simulink subsystem "monocopterChassis"  (R2023a)
settings: Solver=VariableStepAuto  StartTime=0.0  StopTime=100  RelTol=1e-3
undefined symbols (not defined in the file): chassis, fixedStepSize, g
libraries: fl_lib x17, nesl_utility x4
settings Model: DefaultTestHarness=monocopterChassis_Harness1  Creator=imyrsini  LastModifiedBy=imyrsini

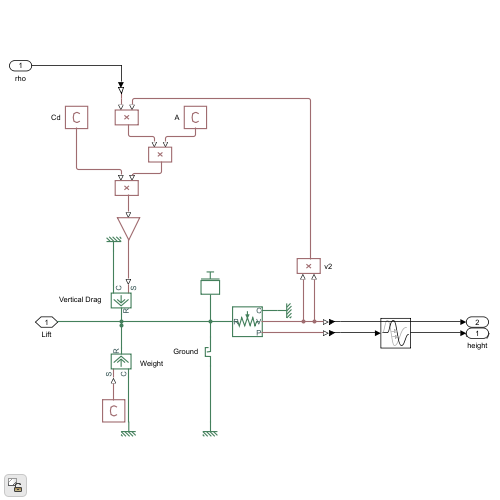
[thumbnail: Simulink's stored preview of the top-level diagram]
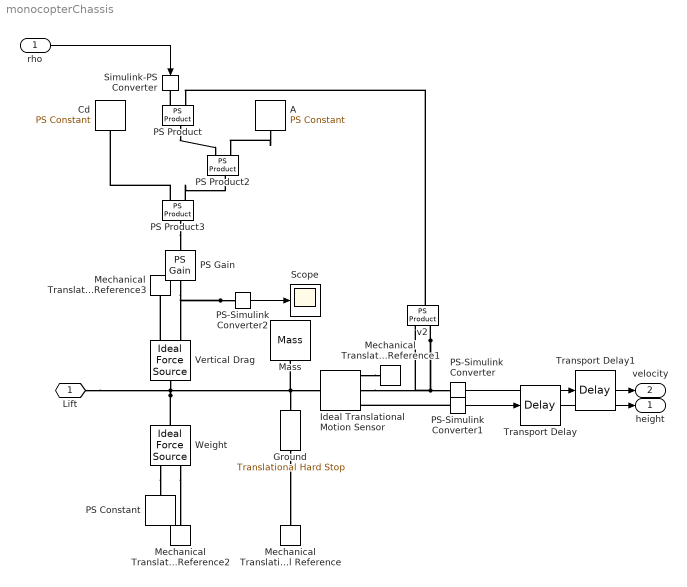
== system monocopterChassis ==
  rho : Inport
  A : fl_lib/Physical Signals/Sources/PS Constant  constant=rotor.area m^2
  Cd : fl_lib/Physical Signals/Sources/PS Constant  constant=2.5
  Ground : fl_lib/Mechanical/Translational Elements/Translational Hard Stop  upper_bnd=inf m  lower_bnd=0 m  model=simscape.enum.hardstop.fullundamped  stiff_up=1e6 N/m  stiff_low=1e12 N/m  D_up=150 N*s/m  D_low=150 N*s/m  transition=0.1 mm  coeff_rest=0.7  v_tol=0.001 m/s  f_tol=0.001 N  x_specify=on  x_priority=High  x=0 m  x_nominal_specify=off  x_nominal_unit=m  x_nominal_value=1  v_specify=off  v_priority=None  v=0 m/s  v_nominal_specify=off  v_nominal_unit=m/s  v_nominal_value=1  f_specify=off  f_priority=None  f=0 N  f_nominal_specify=off  f_nominal_unit=N  f_nominal_value=1  M_specify=off  M_priority=None  M=0
  Ideal Translational Motion Sensor : fl_lib/Mechanical/Mechanical Sensors/Ideal Translational Motion Sensor  reference=foundation.enum.MeasurementReference.difference  acceleration_port=false  velocity_port=true  position_port=true  offset=0 m
  Mass : fl_lib/Mechanical/Translational Elements/Mass  mass=chassis.mass+1000 kg  num_ports=foundation.enum.numPorts2.one  v_specify=off  v_priority=High  v=0 m/s  v_nominal_specify=off  v_nominal_unit=m/s  v_nominal_value=1  f_specify=off  f_priority=None  f=0 N  f_nominal_specify=off  f_nominal_unit=N  f_nominal_value=1
  Mechanical Translational Reference{,1..3} (4 alike) : fl_lib/Mechanical/Translational Elements/Mechanical Translational Reference
  PS Constant : fl_lib/Physical Signals/Sources/PS Constant  constant=-g*chassis.mass N
  PS Gain : fl_lib/Physical Signals/Functions/PS Gain  gain=-1/2
  PS Product : fl_lib/Physical Signals/Functions/PS Product
  PS Product2 : fl_lib/Physical Signals/Functions/PS Product
  PS Product3 : fl_lib/Physical Signals/Functions/PS Product
  PS-Simulink Converter : nesl_utility/PS-Simulink Converter  PhysicalDomain=network_engine_domain  SubClassName=ps_output  LeftPortType=input  RightPortType=output  PseudoPeriodic=off  Frequencies=[]  VectorFormat=inherit  Unit=inherit  AffineConversion=off
  PS-Simulink Converter1 : nesl_utility/PS-Simulink Converter  PhysicalDomain=network_engine_domain  SubClassName=ps_output  LeftPortType=input  RightPortType=output  PseudoPeriodic=off  Frequencies=[]  VectorFormat=inherit  Unit=inherit  AffineConversion=off
  PS-Simulink Converter2 : nesl_utility/PS-Simulink Converter  PhysicalDomain=network_engine_domain  SubClassName=ps_output  LeftPortType=input  RightPortType=output  PseudoPeriodic=off  Frequencies=[]  VectorFormat=inherit  Unit=inherit  AffineConversion=off
  Scope : Scope
  Simulink-PS Converter : nesl_utility/Simulink-PS Converter  PhysicalDomain=network_engine_domain  SubClassName=ps_input  LeftPortType=input  RightPortType=output  PseudoPeriodic=off  Frequencies=[]  NoiseDistribution=none  NoiseParameters=[]  Unit=kg/m^3  AffineConversion=off  FilteringAndDerivatives=provide  SimscapeFilterOrder=1  InputFilterTimeConstant=0.001  UdotUserProvided=0
  Transport Delay : TransportDelay  DelayTime=fixedStepSize
  Transport Delay1 : TransportDelay  DelayTime=fixedStepSize
  Vertical Drag : fl_lib/Mechanical/Mechanical Sources/Ideal Force Source
  Weight : fl_lib/Mechanical/Mechanical Sources/Ideal Force Source
  v2 : fl_lib/Physical Signals/Functions/PS Product
  Lift : PMIOPort  Side=Left
  height : Outport
  velocity : Outport  Port=2
  wires:
  PS-Simulink Converter/1 -> Transport Delay1/1
  rho/1 -> Simulink-PS Converter/1
  PS-Simulink Converter1/1 -> Transport Delay/1
  Transport Delay/1 -> height/1
  Transport Delay1/1 -> velocity/1
  PS-Simulink Converter2/1 -> Scope/1
  connections:
  Vertical Drag/LConn1 -- Ground/LConn1 -- Mass/LConn1 -- Ideal Translational Motion Sensor/LConn1 -- Lift/RConn1 -- Weight/LConn1
  v2/LConn1 -- Ideal Translational Motion Sensor/RConn2 -- v2/LConn2 -- PS-Simulink Converter/LConn1
  PS-Simulink Converter2/LConn1 -- PS Gain/RConn1 -- Vertical Drag/RConn1
  Weight/RConn1 -- PS Constant/RConn1
  Ideal Translational Motion Sensor/RConn1 -- Mechanical Translational Reference1/LConn1
  Ground/RConn1 -- Mechanical Translational Reference/LConn1
  PS-Simulink Converter1/LConn1 -- Ideal Translational Motion Sensor/RConn3
  Vertical Drag/RConn2 -- Mechanical Translational Reference3/LConn1
  Weight/RConn2 -- Mechanical Translational Reference2/LConn1
  PS Product/LConn1 -- Simulink-PS Converter/RConn1
  v2/RConn1 -- PS Product/LConn2
  PS Product/RConn1 -- PS Product2/LConn1
  A/RConn1 -- PS Product2/LConn2
  PS Product3/RConn1 -- PS Gain/LConn1
  PS Product3/LConn2 -- PS Product2/RConn1
  PS Product3/LConn1 -- Cd/RConn1
